simulink model "GFM_SMIB_Scan"  (R2024b)
settings: Solver=FixedStepAuto  StartTime=0  StopTime=200  FixedStep=Ts  RelTol=1e-3
PreLoadFcn:
  | Ts = 2e-5;FS_Frequency=csvread('Frequency_Sweep.csv',1,0); run lpf_param.m;
InitFcn:
  | Ts = 2e-5;FS_Frequency=csvread('Frequency_Sweep.csv',1,0); run lpf_param.m;
StartFcn:
  | Ts = 2e-5;FS_Frequency=csvread('Frequency_Sweep.csv',1,0); run lpf_param.m;
StopFcn:
  | run Bode_Draw.m
values from neighbouring files (symbols this model uses):
  D = zeros(6,4)    [TheoreticalImpedancePlot.m]    (also in TheoreticalImpedancePlotGFL.m = zeros(5,4))
  Fbase = 50    [lpf_param.m]
  fpll = 0.1    [lpf_param.m]
  k_lpf = 0.707    [lpf_param.m]
  wc_lpf = 2*pi*fc_lpf    (= 0.628318530718)    [lpf_param.m]
  x_e = [i_d; i_q; i_d_i; i_q_i; v_d_i; v_q_i; theta; v_dc; v_dc_i; i; i_i; v_lk; p_sum_i; p_lk_i]    [InterlinkAcDcB2B.m]
undefined symbols (not defined in the file or in its folder): ApparatusDiscreDamping, ApparatusPara, ApparatusPowerFlow, ApparatusType, DiscIntNeverNeededParam, OtherInputs, PowerFlow, Wbase, Ybase, Zbase
libraries: SimplusGT x10, discretizing x8, dspindex x4, spsGroundLib x3, spsControlledVoltageSourceLib x3, dspsnks4 x2, simulink x2, spsThreePhaseVIMeasurementLib x2, spsThreePhaseSeriesRLCBranchLib x1, spsThreePhaseParallelRLCBranchLib x1, sps_lib x1
settings Model: Creator=gzhan  LastModifiedBy=gzhan

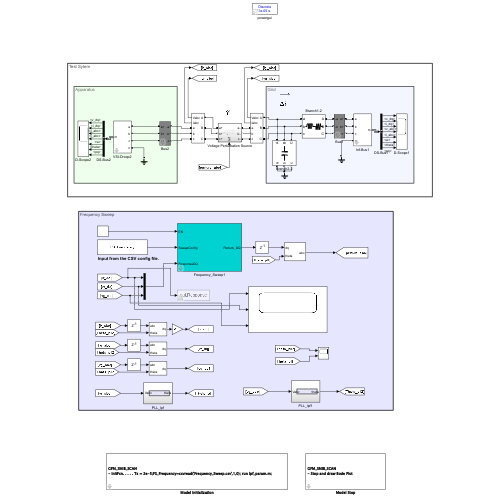
[thumbnail: Simulink's stored preview of the top-level diagram]
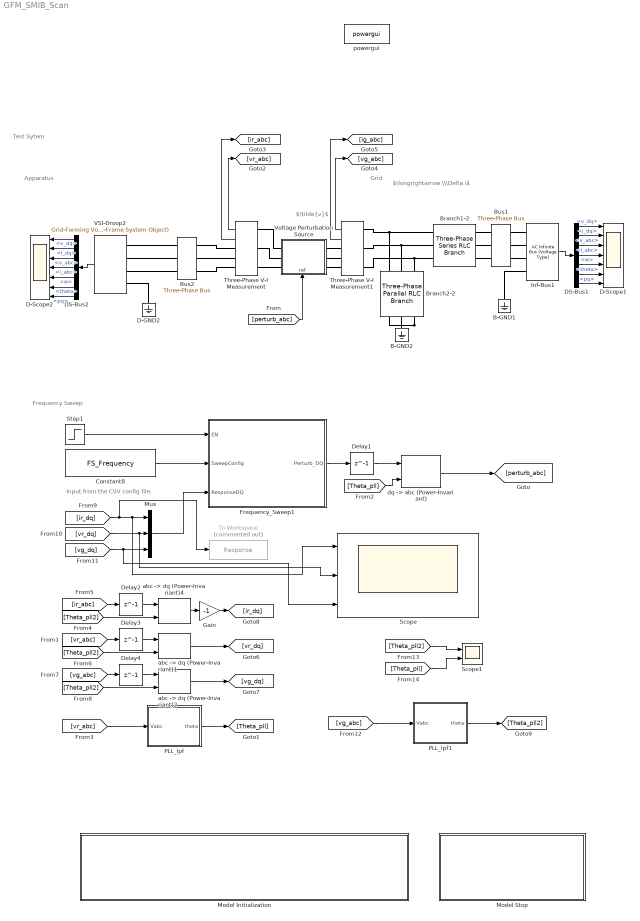
== system GFM_SMIB_Scan ==
  note: $\longrightarrow \\\Delta i$
  note: Test Sytem
  note: Grid
  note: Apparatus
  note: Input from the CSV config file.
  note: Frequency Sweep
  note: $\tilde{v}$
  B-GND1 : spsGroundLib/Ground  LConnTagsString=a
  B-GND2 : spsGroundLib/Ground  LConnTagsString=a
  Branch1-2 : spsThreePhaseSeriesRLCBranchLib/Three-Phase Series RLC Branch  LConnTagsString=A|B|C  RConnTagsString=A|B|C  BranchType=RL  Resistance=(0.02)*Zbase  Inductance=(0.1)*Zbase/Wbase  Capacitance=1e-6  Measurements=None
  Branch2-2 : spsThreePhaseParallelRLCBranchLib/Three-Phase Parallel RLC Branch  LConnTagsString=A|B|C  RConnTagsString=A|B|C  BranchType=C  Resistance=(Inf)*Zbase  Inductance=(Inf)*Zbase/Wbase  Capacitance=(0.02)*Ybase/Wbase  Measurements=None
  Bus1 : SimplusGT/Three-Phase Bus  Vbase=1  Sbase=1
      settings: SourceProductName=Simplus Grid Tool
  Bus2 : SimplusGT/Three-Phase Bus  Vbase=1  Sbase=1
      settings: SourceProductName=Simplus Grid Tool
  Constant8 : Constant  Value=FS_Frequency
  D-GND2 : spsGroundLib/Ground  LConnTagsString=a
  D-Scope1 : Scope  NumInputPorts=7
  D-Scope2 : Scope  NumInputPorts=7
  DS-Bus1 : BusSelector  OutputSignals=v_dq,i_dq,v_abc,i_abc,w,theta,pq
  DS-Bus2 : BusSelector  OutputSignals=v_dq,i_dq,v_abc,i_abc,w,theta,pq
  Delay{1..4} (4 alike) : Delay  DelayLength=1
  Frequency_Sweep1 : Subsystem  mask{Gain=0.02, Interval=1e-2}
      mask prompts: Gain "Output Gain"; Interval "Injection Interval"
  Gain : Gain  Gain=-1
  Inf-Bus1 : SimplusGT/AC Infinite Bus (Voltage Type)  Ts=Ts  Sbase=Sbase  Vbase=Vbase  Wbase=Wbase  vd=PowerFlow{1}(3)  vq=0  theta0=PowerFlow{1}(4)  w=Wbase  R=1e-30
      settings: SourceProductName=Simplus Grid Tool
  Model Initialization : Subsystem  mask(Model Functions){InitFcnVar=Ts = 2e-5;FS_Frequency=csvread('Frequency_Sweep.csv',1,0); run lpf_param.m;}
      mask prompts: InitFcnVar "InitFcn"
      mask init:
      | set_param(bdroot, 'PreLoadFcn', InitFcnVar);
      | set_param(bdroot, 'InitFcn', InitFcnVar);
      | set_param(bdroot, 'StartFcn', InitFcnVar);
      | PLF = get_param(bdroot, 'PreLoadFcn');
      | IF = get_param(bdroot, 'InitFcn');
      | SF = get_param(bdroot, 'StartFcn');
      | 
      | 
      | pos = get_param(gcb, 'Position');
      | width = pos(3) - pos(1); height = pos(4) - pos(2);
      mask Display:
      | text(5, height*0.5, [ ...
      | upper(bdroot) '\n' ...
      | '- InitFcn. . . . . '  get_param(bdroot, 'InitFcn')  ...
      | ], ...
      | 'horizontalAlignment', 'left', 'verticalAlignment', 'middle') ;
  Model Stop : Subsystem  mask(Model Functions){StopFcnVar=run Bode_Draw.m}
      mask prompts: StopFcnVar "StopFcn"
      mask init:
      | set_param(bdroot, 'StopFcn', StopFcnVar);
      | StopF = get_param(bdroot, 'StopFcn');
      | 
      | 
      | pos = get_param(gcb, 'Position');
      | width = pos(3) - pos(1); height = pos(4) - pos(2);
      mask Display:
      | text(5, height*0.5, [ ...
      | upper(bdroot) '\n' ...
      | '- Stop and draw Bode Plot '  ...
      | ], ...
      | 'horizontalAlignment', 'left', 'verticalAlignment', 'middle') ;
  Mux : Mux  Inputs=3
  PLL_lpf : Subsystem
  PLL_lpf1 : Subsystem
  Scope : Scope  NumInputPorts=3
  Scope1 : Scope  NumInputPorts=2
  Step1 : Step  Time=4  SampleTime=0
  Three-Phase V-I Measurement : spsThreePhaseVIMeasurementLib/Three-Phase V-I Measurement  VoltageMeasurement=phase-to-ground  SetLabelV=off  LabelV=Vabc_mea  Vpu=off  VpuLL=off  CurrentMeasurement=yes  SetLabelI=off  LabelI=Iabc_mea  Ipu=off  Pbase=100e6  Vbase=500e3  OutputType=Complex  PhasorSimulation=off  PSBequivalent=0
  Three-Phase V-I Measurement1 : spsThreePhaseVIMeasurementLib/Three-Phase V-I Measurement  VoltageMeasurement=phase-to-ground  SetLabelV=off  LabelV=Vabc_mea  Vpu=off  VpuLL=off  CurrentMeasurement=yes  SetLabelI=off  LabelI=Iabc_mea  Ipu=off  Pbase=100e6  Vbase=500e3  OutputType=Complex  PhasorSimulation=off  PSBequivalent=0
  To Workspace : ToWorkspace  Commented=on  VariableName=Response  SampleTime=-1
  VSI-Droop2 : SimplusGT/Grid-Forming Voltage-Source Inverter (dq-Frame System Object)  Ts=Ts  Sbase=Sbase  Vbase=Vbase  Wbase=Wbase  ApparatusType=ApparatusType{2}  ApparatusPara=ApparatusPara{2}  PowerFlow=ApparatusPowerFlow{2}  x0=x_e{2}  OtherInputs=OtherInputs{2}  DiscreMethod=Hybrid Trapezoidal  EnableInsideModification=off  DiscreDampingFlag=on  DiscreDampingValue=ApparatusDiscreDamping{2}  LinearizationTimes=1  DirectFeedthrough=off
      settings: SourceProductName=Simplus Grid Tool
  Voltage Perturbation Source : Subsystem
      settings: PortSchema="{\"entries\":[{\"content\":{\"sides\":[{\"content\":{\"connectorIds\":[\"LConn1\",\"LConn2\",\"LConn3\"]},\"type\":\"ConnectorPlacement.EquallySpacedRectSide\",\"uuid\":\"6f603e87-6b2e-4585-ad3a-55936445c397\"},{\"content\":{\"connectorIds\":[\"RConn1\",\"RConn2\",\"RConn3\"],\"side\":\"RIGHT\"},\"type\":\"ConnectorPlacement.EquallySpacedRectSide\",\"uuid\":\"08c5aebc-ed45-455a-9198-e657d358a757\"},{\"content\":{\"side\":\"TOP\"},\"type\":\"ConnectorPlacement.EquallySpacedRectSide\",\"uuid\":\"90e892ab-d7d1-4f2e-b125-0b742fd1657c\"},{\"content\":{\"connectorIds\":[\"In1\"],\"side\":\"BOTTOM\"},\"type\":\"ConnectorPlacement.EquallySpacedRectSide\",\"uuid\":\"ba12d237-2ee0-4e5a-b3d4-1de3f90cbef1\"}]},\"type\":\"ConnectorPlacement.EquallySpacedConnector\",\"uuid\":\"0150c08c-ed05-4e99-aa85-f9e708dbbe93\"}],\"packageUris\":[\"http://schema.mathworks.com/mf0/Connector/R2020b\"],\"version\":\"1.0\"}"
  "abc -> dq (Power-Invariant)1" : SimplusGT/abc -> dq (Power-Invariant)  SystemSampleTime=-1  VariantActivationTime=update diagram  AllowFlexibleInterface=on  Latency=0  AutoFrameSizeCalculation=off
      settings: SourceProductName=Simplus Grid Tool
  "abc -> dq (Power-Invariant)2" : SimplusGT/abc -> dq (Power-Invariant)  SystemSampleTime=-1  VariantActivationTime=update diagram  AllowFlexibleInterface=on  Latency=0  AutoFrameSizeCalculation=off
      settings: SourceProductName=Simplus Grid Tool
  "abc -> dq (Power-Invariant)4" : SimplusGT/abc -> dq (Power-Invariant)  SystemSampleTime=-1  VariantActivationTime=update diagram  AllowFlexibleInterface=on  Latency=0  AutoFrameSizeCalculation=off
      settings: SourceProductName=Simplus Grid Tool
  "dq -> abc (Power-Invariant)" : SimplusGT/dq -> abc (Power-Invariant)  SystemSampleTime=-1  VariantActivationTime=update diagram  AllowFlexibleInterface=on  Latency=0  AutoFrameSizeCalculation=off
      settings: SourceProductName=Simplus Grid Tool
  powergui : sps_lib/powergui  Priority=1  SimulationMode=Discrete  SampleTime=Ts  frequency=60  Iterations=50  frequencyindice=0  Pbase=100e6  ErrMax=1e-4  UnitsV=kV  UnitsW=MW  buscounter=0  FunctionMessages=off  echomessages=off  EnableUseOfTLC=off  CurrentSourceSwitches=off  DisableSnubberDevices=off  DisableRonSwitches=off  DisableVfSwitches=off  DisplayEquations=off  AutomaticDiscreteSolvers=off  SolverType=Tustin/Backward Euler (TBE)  Interpol=off  ExternalGateDelay=off  methode=off  Ts=100  x0status=blocks  SPID=on  SwTol=0  HookPort=off  NonlinearTolerance=1e-4  nMaxIteration=100  ContinueOnMaxIteration=off  RestoreLinks=warning  ResistiveCurrentMeasurement=off  Frange=[0:2:500]  Ylog=off  Xlog=on  ShowGrid=off  save=off  variable=ZData  structure=0  ZoomFFT=off  StartTime=0.0  cycles=1  DisplayStyle=1  fundamental=60  FreqAxis=off  MaxFrequency=1000  frequencyindicesteady=1  RmsSteady=1  display=off
  wires:
  Inf-Bus1/1 -> DS-Bus1/1
  DS-Bus1/1 -> D-Scope1/1  "<v_dq>"
  DS-Bus1/2 -> D-Scope1/2  "<i_dq>"
  DS-Bus1/3 -> D-Scope1/3  "<v_abc>"
  DS-Bus1/4 -> D-Scope1/4  "<i_abc>"
  DS-Bus1/5 -> D-Scope1/5  "<w>"
  DS-Bus1/6 -> D-Scope1/6  "<theta>"
  DS-Bus1/7 -> D-Scope1/7  "<pq>"
  VSI-Droop2/1 -> DS-Bus2/1
  DS-Bus2/1 -> D-Scope2/1  "<v_dq>"
  DS-Bus2/2 -> D-Scope2/2  "<i_dq>"
  DS-Bus2/3 -> D-Scope2/3  "<v_abc>"
  DS-Bus2/4 -> D-Scope2/4  "<i_abc>"
  DS-Bus2/5 -> D-Scope2/5  "<w>"
  DS-Bus2/6 -> D-Scope2/6  "<theta>"
  DS-Bus2/7 -> D-Scope2/7  "<pq>"
  "abc -> dq (Power-Invariant)1"/1 -> [vr_dq]
  Gain/1 -> [ir_dq]
  PLL_lpf1/1(theta) -> [Theta_pll2]
  [vr_abc] -> Delay3/1
  [ir_abc] -> Delay2/1
  [Theta_pll] -> "dq -> abc (Power-Invariant)"/2
  Constant8/1 -> Frequency_Sweep1/2(SweepConfig)
  [vg_dq] -> Scope/3, Mux/3
  "abc -> dq (Power-Invariant)4"/1 -> Gain/1
  [Theta_pll2] -> "abc -> dq (Power-Invariant)2"/2
  Frequency_Sweep1/1(Perturb_DQ) -> Delay1/1
  [Theta_pll2] -> "abc -> dq (Power-Invariant)4"/2
  [vr_abc] -> PLL_lpf/1(Vabc)
  PLL_lpf/1(theta) -> [Theta_pll]
  Mux/1 -> Frequency_Sweep1/3(ResponseDQ)
  Step1/1 -> Frequency_Sweep1/1(EN)
  Delay3/1 -> "abc -> dq (Power-Invariant)1"/1
  Delay4/1 -> "abc -> dq (Power-Invariant)2"/1
  [Theta_pll2] -> Scope1/1
  Delay1/1 -> "dq -> abc (Power-Invariant)"/1
  [Theta_pll2] -> "abc -> dq (Power-Invariant)1"/2
  [Theta_pll] -> Scope1/2
  Delay2/1 -> "abc -> dq (Power-Invariant)4"/1
  "abc -> dq (Power-Invariant)2"/1 -> [vg_dq]
  [vr_dq] -> Scope/2, Mux/2
  [vg_abc] -> PLL_lpf1/1(Vabc)
  "dq -> abc (Power-Invariant)"/1 -> [perturb_abc]
  [ir_dq] -> To Workspace/1, Scope/1, Mux/1
  [vg_abc] -> Delay4/1
  Three-Phase V-I Measurement1/1 -> [vg_abc]
  Three-Phase V-I Measurement/1 -> [vr_abc]
  Three-Phase V-I Measurement1/2 -> [ig_abc]
  [perturb_abc] -> Voltage Perturbation Source/1(ref)
  Three-Phase V-I Measurement/2 -> [ir_abc]
  connections:
  B-GND1/LConn1 -- Inf-Bus1/LConn4
  D-GND2/LConn1 -- VSI-Droop2/LConn4
  Bus1/RConn1 -- Branch1-2/LConn1
  Bus1/RConn2 -- Branch1-2/LConn2
  Bus1/RConn3 -- Branch1-2/LConn3
  Inf-Bus1/LConn1 -- Bus1/LConn1
  Inf-Bus1/LConn2 -- Bus1/LConn2
  Inf-Bus1/LConn3 -- Bus1/LConn3
  VSI-Droop2/LConn1 -- Bus2/LConn1
  VSI-Droop2/LConn2 -- Bus2/LConn2
  VSI-Droop2/LConn3 -- Bus2/LConn3
  Branch2-2/RConn3 -- Branch2-2/RConn1 -- B-GND2/LConn1 -- Branch2-2/RConn2
  Bus2/RConn1 -- Three-Phase V-I Measurement/RConn1
  Three-Phase V-I Measurement1/RConn1 -- Voltage Perturbation Source/LConn1
  Three-Phase V-I Measurement1/RConn3 -- Voltage Perturbation Source/LConn3
  Voltage Perturbation Source/RConn1 -- Three-Phase V-I Measurement/LConn1
  Voltage Perturbation Source/RConn3 -- Three-Phase V-I Measurement/LConn3
  Bus2/RConn3 -- Three-Phase V-I Measurement/RConn3
  Bus2/RConn2 -- Three-Phase V-I Measurement/RConn2
  Three-Phase V-I Measurement/LConn2 -- Voltage Perturbation Source/RConn2
  Three-Phase V-I Measurement1/RConn2 -- Voltage Perturbation Source/LConn2
  Three-Phase V-I Measurement1/LConn1 -- Branch1-2/RConn1 -- Branch2-2/LConn1
  Branch1-2/RConn2 -- Branch2-2/LConn2 -- Three-Phase V-I Measurement1/LConn2
  Branch1-2/RConn3 -- Three-Phase V-I Measurement1/LConn3 -- Branch2-2/LConn3

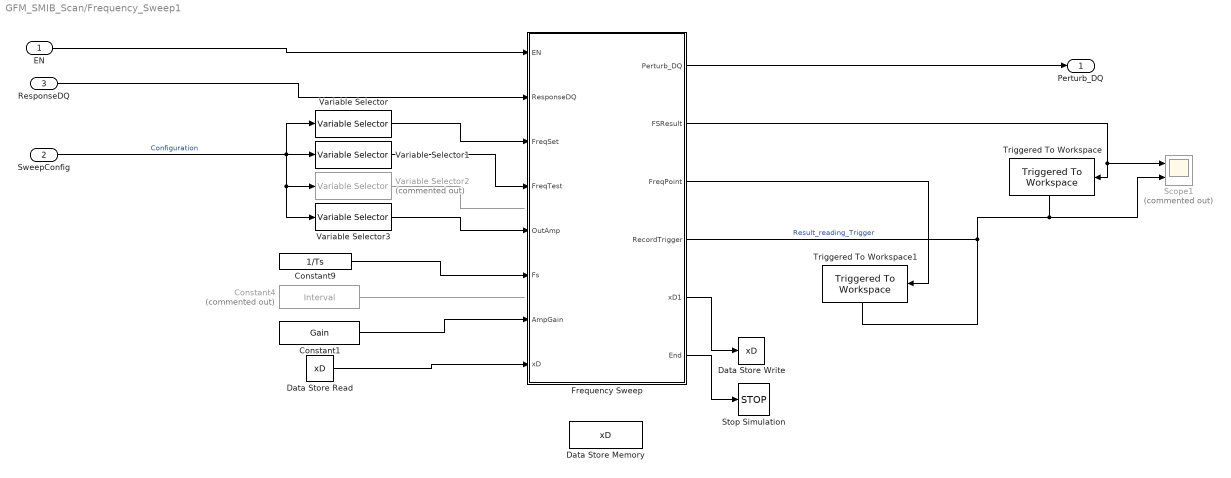
== system GFM_SMIB_Scan/Frequency_Sweep1 ==
  EN : Inport
  SweepConfig : Inport  Port=2
  ResponseDQ : Inport  Port=3
  Constant1 : Constant  Value=Gain
  Constant4 : Constant  Commented=on  Value=Interval
  Constant9 : Constant  Value=1/Ts
  Data Store Memory : DataStoreMemory  DataStoreName=xD  WriteAfterWriteMsg=warning  InitialValue=zeros(57,1)  ShowAdditionalParam=off
  Data Store Read : DataStoreRead  DataStoreName=xD  IndexOptions=Index vector (dialog)  Indices=1  OutputSizes=1
  Data Store Write : DataStoreWrite  DataStoreName=xD  IndexOptions=Index vector (dialog)  Indices=1  OutputSizes=1
  Frequency Sweep : MATLAB Function  TreatAsAtomicUnit=on
  Scope1 : Scope  Commented=on  NumInputPorts=2
  Stop Simulation : Stop
  Triggered To Workspace : dspsnks4/Triggered To Workspace  TriggerType=Rising edge  VariableName=FS_Result  Buffer=5000  Save2DMode=2-D array (concatenate along first dimension)
      settings: FixptAsFi=off
  Triggered To Workspace1 : dspsnks4/Triggered To Workspace  TriggerType=Rising edge  VariableName=FS_Freq_point  Buffer=5000  Save2DMode=2-D array (concatenate along first dimension)
      settings: FixptAsFi=off
  Variable Selector : dspindex/Variable Selector  NumInputs=1  rowsOrCols=Columns  IdxMode=Fixed  Elements=1  ZerOneIdxMode=One-based  errmode=Clip Index  FillMode=on  FillValues=0
  Variable Selector1 : dspindex/Variable Selector  NumInputs=1  rowsOrCols=Columns  IdxMode=Fixed  Elements=2  ZerOneIdxMode=One-based  errmode=Clip Index  FillMode=on  FillValues=0
  Variable Selector2 : dspindex/Variable Selector  Commented=on  NumInputs=1  rowsOrCols=Columns  IdxMode=Fixed  Elements=3  ZerOneIdxMode=One-based  errmode=Clip Index  FillMode=on  FillValues=0
  Variable Selector3 : dspindex/Variable Selector  NumInputs=1  rowsOrCols=Columns  IdxMode=Fixed  Elements=4  ZerOneIdxMode=One-based  errmode=Clip Index  FillMode=on  FillValues=0
  Perturb_DQ : Outport
  wires:
  Variable Selector2/1 -> ?
  Frequency Sweep/2(FSResult) -> Triggered To Workspace/1, Scope1/1
  Frequency Sweep/4(RecordTrigger) -> Triggered To Workspace1/Trigger, Scope1/2, Triggered To Workspace/Trigger  "Result_reading_Trigger"
  Constant4/1 -> ?
  Frequency Sweep/5(xD1) -> Data Store Write/1
  Variable Selector3/1 -> Frequency Sweep/5(OutAmp)
  Variable Selector1/1 -> Frequency Sweep/4(FreqTest)
  SweepConfig/1 -> Variable Selector3/1, Variable Selector2/1, Variable Selector1/1, Variable Selector/1  "Configuration"
  ResponseDQ/1 -> Frequency Sweep/2(ResponseDQ)
  Variable Selector/1 -> Frequency Sweep/3(FreqSet)
  Frequency Sweep/3(FreqPoint) -> Triggered To Workspace1/1
  Data Store Read/1 -> Frequency Sweep/8(xD)
  Constant9/1 -> Frequency Sweep/6(Fs)
  Frequency Sweep/1(Perturb_DQ) -> Perturb_DQ/1
  EN/1 -> Frequency Sweep/1(EN)
  Constant1/1 -> Frequency Sweep/7(AmpGain)
  Frequency Sweep/6(End) -> Stop Simulation/1

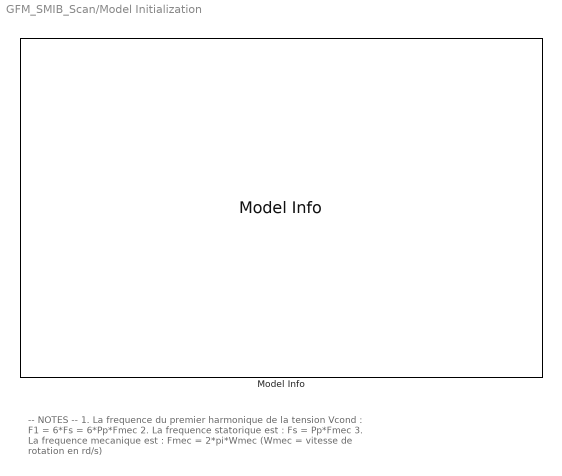
== system GFM_SMIB_Scan/Model Initialization ==
  note: -- NOTES --
      | 1. La frequence du premier harmonique de la tension Vcond :
      |     F1 = 6*Fs = 6*Pp*Fmec
      | 2. La frequence statorique est :
      |     Fs = Pp*Fmec
      | 3. La frequence mecanique est :
      |     Fmec = 2*pi*Wmec  (Wmec = vitesse de rotation en rd/s)
  Model Info : simulink/Model-Wide Utilities/Model Info  Frame=on  DisplayStringWithTags=|  HorizontalTextAlignment=Left  LeftAlignmentValue=0.02
      | - Version <<< %<ModelVersion> >>>
      | 
      | - Description :
      | %<Description>
      | 
      | - Created by :     %<Creator>
      | - Creation date : %<Created>
      | - Modified by :    %<ModifiedBy>
      | - Last modif. :     %<LastModificationDate>

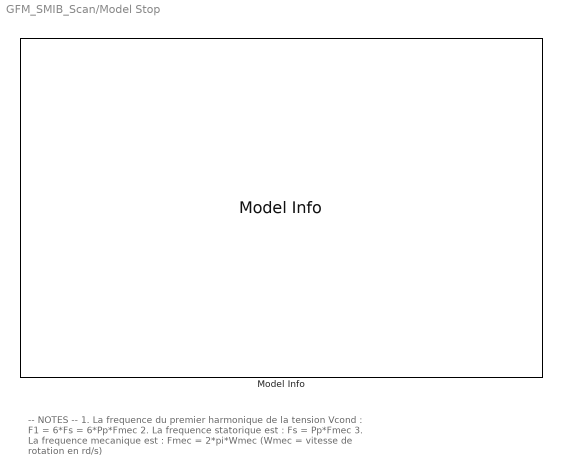
== system GFM_SMIB_Scan/Model Stop ==
  note: -- NOTES --
      | 1. La frequence du premier harmonique de la tension Vcond :
      |     F1 = 6*Fs = 6*Pp*Fmec
      | 2. La frequence statorique est :
      |     Fs = Pp*Fmec
      | 3. La frequence mecanique est :
      |     Fmec = 2*pi*Wmec  (Wmec = vitesse de rotation en rd/s)
  Model Info : simulink/Model-Wide Utilities/Model Info  Frame=on  DisplayStringWithTags=|  HorizontalTextAlignment=Left  LeftAlignmentValue=0.02
      | - Version <<< %<ModelVersion> >>>
      | 
      | - Description :
      | %<Description>
      | 
      | - Created by :     %<Creator>
      | - Creation date : %<Created>
      | - Modified by :    %<ModifiedBy>
      | - Last modif. :     %<LastModificationDate>

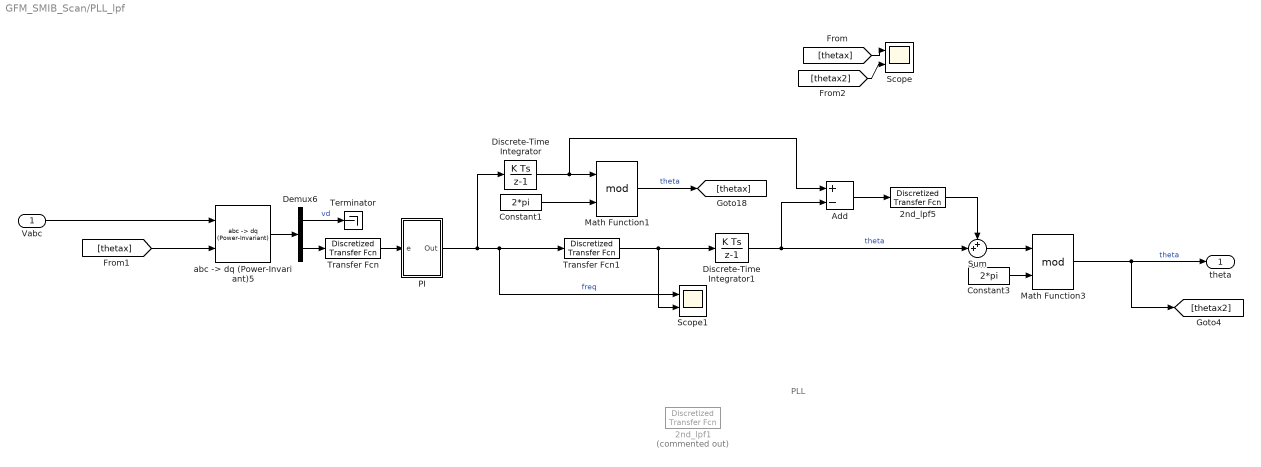
== system GFM_SMIB_Scan/PLL_lpf ==
  note: PLL
  Vabc : Inport
  2nd_lpf1 : discretizing/Discretized Transfer Fcn  Commented=on  Numerator=[wc_lpf^2]  Denominator="[1, 2*k_lpf*wc_lpf,  wc_lpf^2]"  AbsTol=auto  SampleTime=10e-6  method=zoh  Wc=0
  2nd_lpf5 : discretizing/Discretized Transfer Fcn  Numerator=[wc_lpf^2]  Denominator="[1, 2*k_lpf*wc_lpf,  wc_lpf^2]"  AbsTol=auto  SampleTime=Ts  method=zoh  Wc=0
  Add : Sum  Inputs=+-
  Constant1 : Constant  Value=2*pi
  Constant3 : Constant  Value=2*pi
  Demux6 : Demux  Outputs=2
  Discrete-Time Integrator : DiscreteIntegrator  SampleTime=Ts  ICPrevOutput=DiscIntNeverNeededParam  ICPrevScaledInput=DiscIntNeverNeededParam
  Discrete-Time Integrator1 : DiscreteIntegrator  SampleTime=Ts  ICPrevOutput=DiscIntNeverNeededParam  ICPrevScaledInput=DiscIntNeverNeededParam
  Math Function1 : Math  Operator=mod  SignedPower=on
  Math Function3 : Math  Operator=mod  SignedPower=on
  PI : Subsystem  mask{Kp_PLL=2*pi*fpll, Ki_PLL=(2*pi*fpll)^2/4, IntSat_PLL=20000}
      mask prompts: Kp_PLL "Proportional (P)"; Ki_PLL "Integral (I)"; IntSat_PLL "Integrator Saturation Limit"
      mask DialogControl DescGroupVar Prompt: PLL Parameters
  Scope : Scope  NumInputPorts=2
  Scope1 : Scope  NumInputPorts=2
  Sum : Sum  Inputs=++|
  Terminator : Terminator
  Transfer Fcn : discretizing/Discretized Transfer Fcn  Numerator=[1]  Denominator=[1/(2*pi*50) 1]  AbsTol=auto  SampleTime=Ts  method=zoh  Wc=0
  Transfer Fcn1 : discretizing/Discretized Transfer Fcn  Numerator=[1]  Denominator=[1/(2*pi*1) 1]  AbsTol=auto  SampleTime=Ts  method=zoh  Wc=0
  "abc -> dq (Power-Invariant)5" : SimplusGT/abc -> dq (Power-Invariant)  SystemSampleTime=-1  VariantActivationTime=update diagram  AllowFlexibleInterface=on  Latency=0  AutoFrameSizeCalculation=off
      settings: SourceProductName=Simplus Grid Tool
  theta : Outport
  wires:
  Math Function3/1 -> theta/1, [thetax2]  "theta"
  Discrete-Time Integrator1/1 -> Sum/2, Add/2  "theta"
  Constant1/1 -> Math Function1/2
  Transfer Fcn/1 -> PI/1(e)
  Math Function1/1 -> [thetax]  "theta"
  Sum/1 -> Math Function3/1
  Transfer Fcn1/1 -> Scope1/2, Discrete-Time Integrator1/1
  Constant3/1 -> Math Function3/2
  [thetax] -> "abc -> dq (Power-Invariant)5"/2
  Demux6/2 -> Transfer Fcn/1
  PI/1(Out) -> Transfer Fcn1/1, Scope1/1, Discrete-Time Integrator/1  "freq"
  "abc -> dq (Power-Invariant)5"/1 -> Demux6/1
  Add/1 -> 2nd_lpf5/1
  Demux6/1 -> Terminator/1  "vd"
  Vabc/1 -> "abc -> dq (Power-Invariant)5"/1
  Discrete-Time Integrator/1 -> Add/1, Math Function1/1
  [thetax] -> Scope/1
  [thetax2] -> Scope/2
  2nd_lpf5/1 -> Sum/1

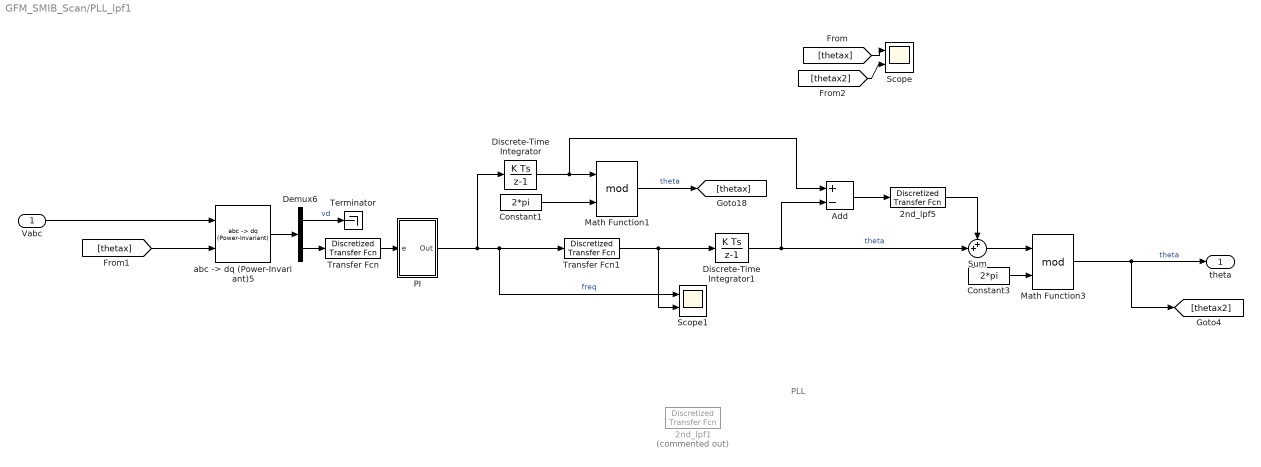
== system GFM_SMIB_Scan/PLL_lpf1 ==
  note: PLL
  Vabc : Inport
  2nd_lpf1 : discretizing/Discretized Transfer Fcn  Commented=on  Numerator=[wc_lpf^2]  Denominator="[1, 2*k_lpf*wc_lpf,  wc_lpf^2]"  AbsTol=auto  SampleTime=10e-6  method=zoh  Wc=0
  2nd_lpf5 : discretizing/Discretized Transfer Fcn  Numerator=[wc_lpf^2]  Denominator="[1, 2*k_lpf*wc_lpf,  wc_lpf^2]"  AbsTol=auto  SampleTime=Ts  method=zoh  Wc=0
  Add : Sum  Inputs=+-
  Constant1 : Constant  Value=2*pi
  Constant3 : Constant  Value=2*pi
  Demux6 : Demux  Outputs=2
  Discrete-Time Integrator : DiscreteIntegrator  SampleTime=Ts  ICPrevOutput=DiscIntNeverNeededParam  ICPrevScaledInput=DiscIntNeverNeededParam
  Discrete-Time Integrator1 : DiscreteIntegrator  SampleTime=Ts  ICPrevOutput=DiscIntNeverNeededParam  ICPrevScaledInput=DiscIntNeverNeededParam
  Math Function1 : Math  Operator=mod  SignedPower=on
  Math Function3 : Math  Operator=mod  SignedPower=on
  PI : Subsystem  mask{Kp_PLL=2*pi*fpll, Ki_PLL=(2*pi*fpll)^2/4, IntSat_PLL=20000}
      mask prompts: Kp_PLL "Proportional (P)"; Ki_PLL "Integral (I)"; IntSat_PLL "Integrator Saturation Limit"
      mask DialogControl DescGroupVar Prompt: PLL Parameters
  Scope : Scope  NumInputPorts=2
  Scope1 : Scope  NumInputPorts=2
  Sum : Sum  Inputs=++|
  Terminator : Terminator
  Transfer Fcn : discretizing/Discretized Transfer Fcn  Numerator=[1]  Denominator=[1/(2*pi*50) 1]  AbsTol=auto  SampleTime=Ts  method=zoh  Wc=0
  Transfer Fcn1 : discretizing/Discretized Transfer Fcn  Numerator=[1]  Denominator=[1/(2*pi*1) 1]  AbsTol=auto  SampleTime=Ts  method=zoh  Wc=0
  "abc -> dq (Power-Invariant)5" : SimplusGT/abc -> dq (Power-Invariant)  SystemSampleTime=-1  VariantActivationTime=update diagram  AllowFlexibleInterface=on  Latency=0  AutoFrameSizeCalculation=off
      settings: SourceProductName=Simplus Grid Tool
  theta : Outport
  wires:
  Math Function3/1 -> theta/1, [thetax2]  "theta"
  Discrete-Time Integrator1/1 -> Sum/2, Add/2  "theta"
  Constant1/1 -> Math Function1/2
  Transfer Fcn/1 -> PI/1(e)
  Math Function1/1 -> [thetax]  "theta"
  Sum/1 -> Math Function3/1
  Transfer Fcn1/1 -> Scope1/2, Discrete-Time Integrator1/1
  Constant3/1 -> Math Function3/2
  [thetax] -> "abc -> dq (Power-Invariant)5"/2
  Demux6/2 -> Transfer Fcn/1
  PI/1(Out) -> Transfer Fcn1/1, Scope1/1, Discrete-Time Integrator/1  "freq"
  "abc -> dq (Power-Invariant)5"/1 -> Demux6/1
  Add/1 -> 2nd_lpf5/1
  Demux6/1 -> Terminator/1  "vd"
  Vabc/1 -> "abc -> dq (Power-Invariant)5"/1
  Discrete-Time Integrator/1 -> Add/1, Math Function1/1
  [thetax] -> Scope/1
  [thetax2] -> Scope/2
  2nd_lpf5/1 -> Sum/1

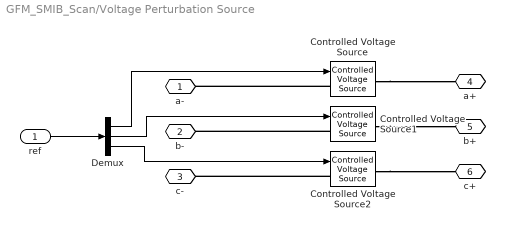
== system GFM_SMIB_Scan/Voltage Perturbation Source ==
  ref : Inport
  Controlled Voltage Source : spsControlledVoltageSourceLib/Controlled Voltage Source  Initialize=on  Source_Type=AC  Amplitude=0  Phase=0  Frequency=0  Measurements=None
  Controlled Voltage Source1 : spsControlledVoltageSourceLib/Controlled Voltage Source  Initialize=on  Source_Type=AC  Amplitude=0  Phase=0  Frequency=0  Measurements=None
  Controlled Voltage Source2 : spsControlledVoltageSourceLib/Controlled Voltage Source  Initialize=on  Source_Type=AC  Amplitude=0  Phase=0  Frequency=0  Measurements=None
  Demux : Demux  Outputs=3
  a- : PMIOPort  Side=Left
  b- : PMIOPort  Port=2  Side=Left
  c- : PMIOPort  Port=3  Side=Left
  a+ : PMIOPort  Port=4  Side=Right
  b+ : PMIOPort  Port=5  Side=Right
  c+ : PMIOPort  Port=6  Side=Right
  wires:
  Demux/2 -> Controlled Voltage Source1/1
  Demux/3 -> Controlled Voltage Source2/1
  ref/1 -> Demux/1
  Demux/1 -> Controlled Voltage Source/1
  connections:
  Controlled Voltage Source/LConn1 -- a-/RConn1
  Controlled Voltage Source1/RConn1 -- b+/RConn1
  Controlled Voltage Source1/LConn1 -- b-/RConn1
  Controlled Voltage Source/RConn1 -- a+/RConn1
  Controlled Voltage Source2/RConn1 -- c+/RConn1
  Controlled Voltage Source2/LConn1 -- c-/RConn1

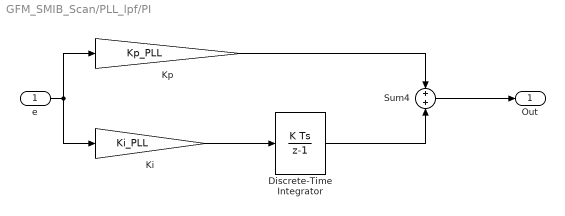
== system GFM_SMIB_Scan/PLL_lpf/PI ==
  e : Inport
  Discrete-Time Integrator : DiscreteIntegrator  gainval=1  InitialCondition=2*pi*Fbase  SampleTime=Ts  LimitOutput=on  UpperSaturationLimit=2*pi*Fbase + IntSat_PLL  LowerSaturationLimit=2*pi*Fbase - IntSat_PLL  ICPrevOutput=DiscIntNeverNeededParam  ICPrevScaledInput=DiscIntNeverNeededParam
  Ki : Gain  Gain=Ki_PLL  SaturateOnIntegerOverflow=on  OutDataTypeStr=Inherit: Same as input  ParamDataTypeStr=Inherit: Same as input
  Kp : Gain  Gain=Kp_PLL  SaturateOnIntegerOverflow=on  OutDataTypeStr=Inherit: Same as input  ParamDataTypeStr=Inherit: Same as input
  Sum4 : Sum  SaturateOnIntegerOverflow=on
  Out : Outport
  wires:
  Sum4/1 -> Out/1
  Discrete-Time Integrator/1 -> Sum4/2
  e/1 -> Kp/1, Ki/1
  Kp/1 -> Sum4/1
  Ki/1 -> Discrete-Time Integrator/1

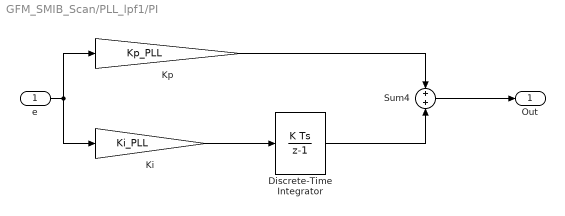
== system GFM_SMIB_Scan/PLL_lpf1/PI ==
  e : Inport
  Discrete-Time Integrator : DiscreteIntegrator  gainval=1  InitialCondition=2*pi*Fbase  SampleTime=Ts  LimitOutput=on  UpperSaturationLimit=2*pi*Fbase + IntSat_PLL  LowerSaturationLimit=2*pi*Fbase - IntSat_PLL  ICPrevOutput=DiscIntNeverNeededParam  ICPrevScaledInput=DiscIntNeverNeededParam
  Ki : Gain  Gain=Ki_PLL  SaturateOnIntegerOverflow=on  OutDataTypeStr=Inherit: Same as input  ParamDataTypeStr=Inherit: Same as input
  Kp : Gain  Gain=Kp_PLL  SaturateOnIntegerOverflow=on  OutDataTypeStr=Inherit: Same as input  ParamDataTypeStr=Inherit: Same as input
  Sum4 : Sum  SaturateOnIntegerOverflow=on
  Out : Outport
  wires:
  Sum4/1 -> Out/1
  Discrete-Time Integrator/1 -> Sum4/2
  e/1 -> Kp/1, Ki/1
  Kp/1 -> Sum4/1
  Ki/1 -> Discrete-Time Integrator/1

== matlab function GFM_SMIB_Scan/Frequency_Sweep1/Frequency Sweep ==
  data: EN input; Perturb_DQ output; ResponseDQ input size=[1 6]; FreqSet input; FreqTest input; OutAmp input; Fs input; AmpGain input; xD input; FSResult output; FreqPoint output; RecordTrigger output; xD1 output; End output
function [Perturb_DQ, FSResult, FreqPoint, RecordTrigger, xD1, End] = fcn(EN,ResponseDQ, FreqSet, FreqTest, OutAmp, Fs, AmpGain, xD)
% This function performs online frequency scanning using a state machine. 
%   - D and Q axis perturbations at specified frequencies
%   - The system response measured (Voltage and Currents)
%   - System admittance, Apparatus Admittance and Grid admittance are
%   calculated
% This current version uses a fixed window to detect whether steady state
% has been reached for each frequency point.
%
% Inputs:
%   EN          : Enable signal (1 to run, 0 to reset)
%   ResponseDQ  : 1x6 vector of system responses [ID, IQ, VAD, VAQ, VGD, VGQ]
%   FreqSet     : Vector of frequencies to apply perturbation (Hz)
%   FreqTest    : Vector of frequencies to analyze (DFT) (Hz)
%   OutAmp      : Vector of perturbation amplitudes for each frequency
%   Fs          : Sampling frequency (Hz)
%   AmpGain     : Global gain for perturbation amplitude
%   xD          : State vector (storage between calls)
%
% Outputs:
%   Perturb_DQ    : [OutVD, OutVQ] perturbation signal to inject
%   FSResult      : 2x6 complex vector of 2x2 admittances [Ysys, YA, YG]
%   FreqPoint     : The current frequency being tested
%   RecordTrigger : A one-sample pulse (==1) when a new result is calculated
%   xD1           : Updated state vector for the next time step
%   End           : Boolean Simulation End 
%
% ------------------- Tuning: Steady-state detector ---------------------- %
% These parameters control the sensitivity and speed of the steady-state detector.
MIN_CYCLES_WINDOWS = 1;    % always do at least one full test cycle before checking
MAX_CYCLES_WINDOWS = 20;   % safety cap to avoid hanging if state never stabilizes
TOL_MAG    = 1e-3;         % relative magnitude tolerance for steady-state (0.1%)
TOL_PHASE  = 1*pi/180;     % phase tolerance (radians) (~1 deg)
STABLE_K   = 1;            % consecutive stable cycles required to confirm steady state
EPS        = 1e-12;        % small number to prevent division by zero
CYCLES = 3;                % number of cycles to use for each fixed DFT window
% -------------------Initialise Outputs-----------------------------------%
% Pre-allocate output matrices for admittances
YA        = complex(zeros(2,2)); % Admittance YA = -I / VA
YG        = complex(zeros(2,2)); % Admittance YG = I / VG
Ysys      = complex(zeros(2,2)); % System Admittance Ysys = I / V_perturb
FSResult  = complex(zeros(2,6)); % Final result matrix [Ysys, YA, YG]
RecordTrigger = 0;               % Output trigger pulse
End = 0;                         % Simulation End Boolean
% ------------------- Read States ----------------------------------------%
% 'xD' stores the function's internal state between simulation steps.
CaseK = xD(1);    % Current state in the state machine (0, 1, 2, 3, 9)
Ns    = xD(2);    % Number of samples for perturbation signal generation
Nt    = xD(3);    % Number of samples for DFT analysis window
n     = xD(4);    % Current sample counter within a window (1 to Nt)
kc    = xD(5);    % Current frequency index (points to FreqSet(kc))
OutVD = xD(6);    % Current D-axis perturbation output
OutVQ = xD(7);    % Current Q-axis perturbation output
% Sums for DFT accumulation [ID, IQ, VAD, VAQ, VGD, VGQ]
% These are complex accumulators for the 6 response signals.
Sum = complex([xD(8)+1i*xD(9),  xD(10)+1i*xD(11), ...
               xD(20)+1i*xD(21), xD(22)+1i*xD(23), ...
               xD(32)+1i*xD(33), xD(34)+1i*xD(35)]);
% Final DFT results after D-axis sweep [ID, IQ, VAD, VAQ, VGD, VGQ]
FinalD = complex([xD(12)+1i*xD(13),  xD(14)+1i*xD(15), ...
                  xD(24)+1i*xD(25),  xD(26)+1i*xD(27), ...
                  xD(36)+1i*xD(37),  xD(38)+1i*xD(39)]).'; % Transpose to 6x1
% Final DFT results after Q-axis sweep [ID, IQ, VAD, VAQ, VGD, VGQ]
FinalQ = complex([xD(16)+1i*xD(17),  xD(18)+1i*xD(19), ...
                  xD(28)+1i*xD(29),  xD(30)+1i*xD(31), ...
                  xD(40)+1i*xD(41),  xD(42)+1i*xD(43)]).'; % Transpose to 6x1
% --- Legacy TWait(44) removed ---
% Steady-state detector states (shifted down by 1)
cycCount     = xD(44);     % Number of test cycles completed at this frequency
stableCount  = xD(45);     % Number of consecutive stable cycles
PrevRe       = [xD(46) xD(47) xD(48) xD(49) xD(50) xD(51)]; % Real part of previous DFT
PrevIm       = [xD(52) xD(53) xD(54) xD(55) xD(56) xD(57)]; % Imag part of previous DFT
Prev         = complex(PrevRe(:), PrevIm(:));   % 6x1 complex vector of previous DFT results
% Get total number of frequencies to test
FrequencyNum = numel(FreqSet);
% --- Safety Check ---
% Ensure gain is not zero, which would cause division by zero later
if AmpGain==0 || (kc>=1 && kc<=FrequencyNum && OutAmp(kc)==0)
    error('AmpGain and OutAmp(kc) must be non-zero');
end
% Reshape response input to a 1x6 row vector for easier matrix math
Resp = reshape(ResponseDQ,1,6);
%% Main Loop
if EN==0
    % If Enable is low, reset the perturbation outputs
    OutVD=0;
    OutVQ=0;
    % Note: State variables are NOT reset here, they are reset in Case 0
    % when EN goes high.
else
    % --- State Machine ---
    switch CaseK
        case 0  % State 0: Initialization
            RecordTrigger = 0; % Ensure trigger is low
            kc = 1;            % Start with the first frequency
            CaseK = 1;         % Move to setup state
        case 1  % State 1: Setup for new frequency
            if kc > FrequencyNum
                % If frequency index is past the end of the list, sweep is done
                OutVD=0; OutVQ=0; % Turn off perturbation
                CaseK = 9;       % Move to 'finished' state
            else
                % --- Prepare for a new frequency sweep ---
                Sum(:)=0;  % Reset DFT accumulators
                % Calculate number of samples for perturbation generation (Ns)
                % and DFT analysis (Nt) based on Fs, Freq, and CYCLES
                Ns = max(1, round(Fs/FreqSet(kc)*CYCLES));
                Nt = max(1, round(Fs/FreqTest(kc)*CYCLES));
                OutVD=0; OutVQ=0; % Ensure perturbation is off during setup
                n = 1;            % Reset sample counter
                % Reset steady-state detector variables
                cycCount = 0;
                stableCount = 0;
                Prev(:) = 0;
                CaseK = 2;         % Move to D-axis perturbation state
            end
        case 2   % State 2: D-axis perturbation and analysis
            % Generate D-axis sinusoidal perturbation
            OutVD = OutAmp(kc)*sin(2*pi*CYCLES*n/Ns)*AmpGain;
            OutVQ = 0;
            % Calculate DFT complex phasor for this sample
            ang = 2*pi*CYCLES*(n-1)/Nt;
            ph  = sin(ang) + 1i*cos(ang);
            % Accumulate the DFT sum (dot product of response and phasor)
            Sum = Sum + Resp * ph;
            if n < Nt
                % If window is not full, increment sample counter
                n = n + 1;
            else
                % --- One test cycle completed on D-axis ---
                % Scale the accumulated sum to get the DFT phasor
                scale  = 2*FreqSet(kc)/CYCLES/Fs; % DFT scaling factor
                Curr   = scale*Sum.';     % 6x1 complex phasor result
                if cycCount >= 1
                    % --- Steady-State Check (if not the first cycle) ---
                    % Compare current result (Curr) vs. previous (Prev)
                    % Calculate relative magnitude difference
                    dmag   = abs(abs(Curr) - abs(Prev)) ./ max(abs(Curr), EPS);
                    % Calculate phase difference
                    dphase = angle(Curr) - angle(Prev);
                    % Wrap phase difference to [-pi, pi]
                    dphase = atan2(sin(dphase), cos(dphase));
                    % Check if all 6 signals are stable within tolerance
                    isStable = all(dmag <= TOL_MAG) && all(abs(dphase) <= TOL_PHASE);
                    if isStable
                        stableCount = stableCount + 1; % Increment stable counter
                    else
                        stableCount = 0; % Reset if any signal is unstable
                    end
                end
                Prev      = Curr;         % Store current result for next comparison
                cycCount  = cycCount + 1; % Increment total cycle counter
                % --- Decision: Move on or repeat? ---
                if (cycCount >= MIN_CYCLES_WINDOWS && stableCount >= STABLE_K) || (cycCount >= MAX_CYCLES_WINDOWS)
                    % Condition 1: Min cycles done AND stable count reached
                    % Condition 2: Max cycles limit reached
                    
                    % Accept this result as steady-state for D-axis
                    FinalD = Prev;
                    % Prepare for Q-axis sweep
                    Sum(:) = 0; n = 1; % Reset accumulators and counter
                    cycCount = 0; stableCount = 0; % Reset detector
                    Prev(:)  = 0;
                    CaseK = 3;         % Move to Q-axis state
                else
                    % Not stable yet, run another test cycle
                    Sum(:) = 0; n = 1;   % Reset for another D-axis cycle
                    % Stay in CaseK = 2
                end
            end
        case 3   % State 3: Q-axis perturbation and analysis
            % This state is analogous to Case 2, but for the Q-axis.
            OutVD = 0;
            OutVQ = OutAmp(kc)*sin(2*pi*CYCLES*n/Ns)*AmpGain;
            % Calculate DFT complex phasor
            ang = 2*pi*CYCLES*(n-1)/Nt;
            ph  = sin(ang) + 1i*cos(ang);
            % Accumulate DFT sum
            Sum = Sum + Resp * ph;
            if n < Nt
                % If window is not full, increment sample counter
                n = n + 1;
            else
                % --- One test cycle completed on Q-axis ---
                scale  = 2*FreqSet(kc)/CYCLES/Fs; % DFT scaling
                Curr   = scale*Sum.';     % 6x1 complex phasor
                % --- Steady-State Check ---
                if cycCount >= 1
                    dmag   = abs(abs(Curr) - abs(Prev)) ./ max(abs(Curr), EPS);
                    dphase = angle(Curr) - angle(Prev);
                    dphase = atan2(sin(dphase), cos(dphase));
                    isStable = all(dmag <= TOL_MAG) && all(abs(dphase) <= TOL_PHASE);
                    if isStable
                        stableCount = stableCount + 1;
                    else
                        stableCount = 0;
                    end
                end
                Prev      = Curr;
                cycCount  = cycCount + 1;
                % --- Decision: Finalize or repeat? ---
                if (cycCount >= MIN_CYCLES_WINDOWS && stableCount >= STABLE_K) || (cycCount >= MAX_CYCLES_WINDOWS)
                    % Steady state reached for Q-axis
                    FinalQ = Prev;
                    % --- Calculate Admittances ---
                    % Build 2x2 matrices from the 6x1 D and Q result vectors
                    % I = [I_d_from_Vd, I_d_from_Vq; I_q_from_Vd, I_q_from_Vq]
                    I  = [FinalD(1), FinalQ(1);  FinalD(2), FinalQ(2)];
                    VA = [FinalD(3), FinalQ(3);  FinalD(4), FinalQ(4)];
                    VG = [FinalD(5), FinalQ(5);  FinalD(6), FinalQ(6)];
                    % Calculate admittance matrices using pseudo-inverse (pinv)
                    % for numerical stability.
                    % Y = I * V^-1
                    YA  = -I * pinv(VA);  % Note the negative sign
                    YG  = I * pinv(VG);
                    
                    % Ysys is calculated relative to the known perturbation amplitude
                    % V_perturb = [Amp, 0; 0, Amp] (assuming same D/Q amp)
                    % Ysys = I * V_perturb^-1
                    Ysys = -I/(OutAmp(kc)*AmpGain);
                    % Set trigger pulse high for one sample
                    RecordTrigger = 1;
                    
                    % --- Advance to next frequency ---
                    kc = kc + 1;
                    if kc > FrequencyNum
                        % Finished all frequencies
                        CaseK = 9;
                    else
                        % Prepare for next frequency
                        Sum(:)=0; n=1; cycCount=0; stableCount=0; Prev(:)=0;
                        CaseK = 1; % Go back to setup state
                    end
                else
                    % Not stable, run another Q-axis test cycle
                    Sum(:) = 0; n = 1;
                    % Stay in CaseK = 3
                end
            end
        case 9  % State 9: Finished
            % Sweep is complete. Hold outputs at 0.
            OutVD=0;
            OutVQ=0;
            % The state machine will stay here until EN=0.
    end
end
%% Set Outputs
% Pack all internal states back into the 'xD1' state vector
% This ensures they are saved for the next function call.

xD1 = zeros(1,57);   % Initialize output state vector (new length 57)
xD1(1:7)   = [CaseK, Ns, Nt, n, kc, OutVD, OutVQ]; % Main states

% Pack DFT sums (complex -> 2 reals)
xD1(8:11)  = [real(Sum(1)), imag(Sum(1)), real(Sum(2)), imag(Sum(2))]; % ID, IQ
xD1(20:23) = [real(Sum(3)), imag(Sum(3)), real(Sum(4)), imag(Sum(4))]; % VAD, VAQ
xD1(32:35) = [real(Sum(5)), imag(Sum(5)), real(Sum(6)), imag(Sum(6))]; % VGD, VGQ

% Pack Final D-axis results
xD1(12:15) = [real(FinalD(1)), imag(FinalD(1)), real(FinalD(2)), imag(FinalD(2))];
xD1(24:27) = [real(FinalD(3)), imag(FinalD(3)), real(FinalD(4)), imag(FinalD(4))];
xD1(36:39) = [real(FinalD(5)), imag(FinalD(5)), real(FinalD(6)), imag(FinalD(6))];

% Pack Final Q-axis results
xD1(16:19) = [real(FinalQ(1)), imag(FinalQ(1)), real(FinalQ(2)), imag(FinalQ(2))];
xD1(28:31) = [real(FinalQ(3)), imag(FinalQ(3)), real(FinalQ(4)), imag(FinalQ(4))];
xD1(40:43) = [real(FinalQ(5)), imag(FinalQ(5)), real(FinalQ(6)), imag(FinalQ(6))];

% --- TWait(44) removed, states shifted ---
% Pack steady-state detector states
xD1(44) = cycCount;
xD1(45) = stableCount;
xD1(46:51) = real(Prev).';   % 6 real parts
xD1(52:57) = imag(Prev).';   % 6 imaginary parts

% --- Assign final function outputs ---
Perturb_DQ = [OutVD, OutVQ]; % Perturbation signal
if kc>0 && EN==1
    % Reshape 2x2 matrices into a 2x6 complex row vector for output
    FSResult = [Ysys, YA, YG];
    
    % Decide which frequency index to report:
    % - When RecordTrigger==1, a result for the *previous* kc was just finalized,
    %   but kc has already been incremented. Report kc-1 in that case.
    % - Otherwise, report the current kc being processed.
    if RecordTrigger==1
        idx = kc - 1;
    else
        idx = kc;
    end

    % Clamp idx to valid range [1, FrequencyNum]
    if FrequencyNum >= 1
        idx = max(1, min(idx, FrequencyNum));
        FreqPoint = FreqSet(idx);
    else
        FreqPoint = 0;
    end
    End = double(CaseK==9);
else
    % If disabled or not started, output zeros
    FSResult(:) = 0;
    FreqPoint   = 0;
    End         = 0;             
end
end
